simulink model "Closed_loop_Practical_BPS_LQR_Controller"  (R2023b)
settings: Solver=VariableStepAuto  StartTime=0.0  StopTime=10  RelTol=1e-3
undefined symbols (not defined in the file): A, B, C, Continuous, D, Discrete, Ke, Kr, Time
libraries: ctrlSharedLib x2, simulink_extras x1, simulink x1
settings Model: Creator=msdbg  LastModifiedBy=msdbg

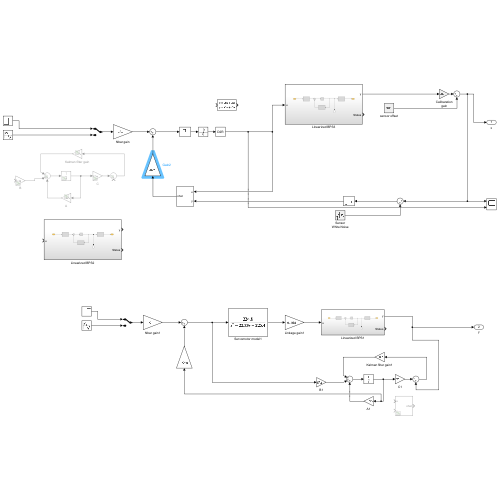
[thumbnail: Simulink's stored preview of the top-level diagram]
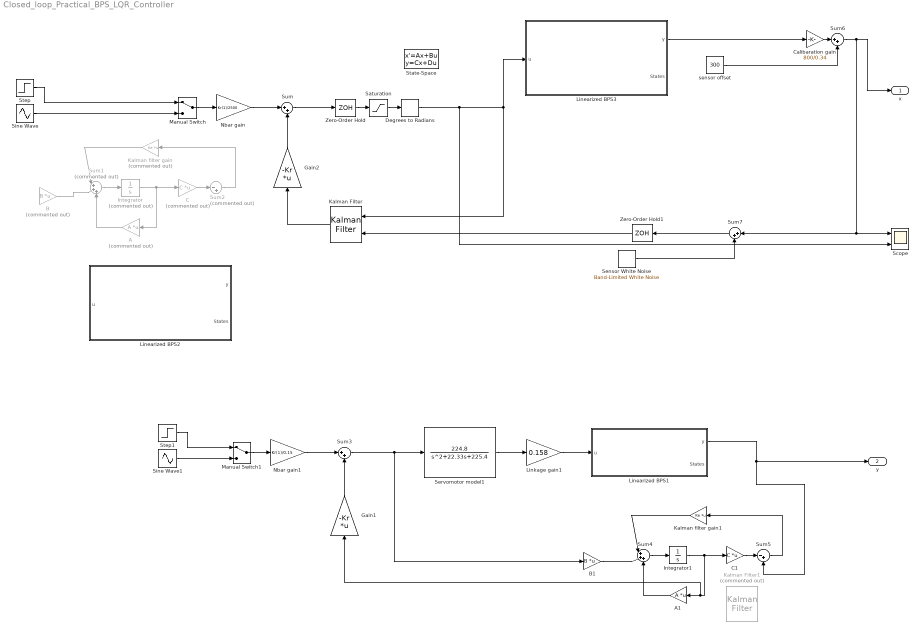
== system Closed_loop_Practical_BPS_LQR_Controller ==
  A : Gain  Commented=on  Gain=A  Multiplication=Matrix(K*u)
  A1 : Gain  Gain=A  Multiplication=Matrix(K*u)
  B : Gain  Commented=on  Gain=B  Multiplication=Matrix(K*u)
  B1 : Gain  Gain=B  Multiplication=Matrix(K*u)
  C : Gain  Commented=on  Gain=C  Multiplication=Matrix(K*u)
  C1 : Gain  Gain=C  Multiplication=Matrix(K*u)
  Calibaration gain : Gain  Gain=800/0.34
  Degrees to Radians : simulink_extras/Transformations/Degrees to Radians
  Gain1 : Gain  Gain=-Kr  Multiplication=Matrix(K*u)
  Gain2 : Gain  Gain=-Kr  Multiplication=Matrix(K*u)
  Integrator : Integrator  Commented=on
  Integrator1 : Integrator
  Kalman Filter : ctrlSharedLib/Kalman Filter  TimeDomain=Discrete-Time  UseCurrentEstimator=on  ModelSource=LTI State-Space Variable  ModelSourceVariable=DBPS  A=A  B=B  C=C  D=D  NumberOfStates=1  NumberOfInputs=1  NumberOfOutputs=1  InitialEstimateSource=Dialog  X0=0  P0=10  UseK=off  UseGH=off  NumberOfProcessNoiseInputs=1  G=1  TimeInvariantG=on  H=0  TimeInvariantH=on  Q=w  TimeInvariantQ=on  R=0.01  TimeInvariantR=on  N=0  TimeInvariantN=on  AddInputPort=on  AddEnablePort=off  OutputEstimatedY=off  OutputP=off  Ts=0.05
  Kalman Filter1 : ctrlSharedLib/Kalman Filter  Commented=on  TimeDomain=Continuous-Time  UseCurrentEstimator=on  ModelSource=LTI State-Space Variable  ModelSourceVariable=BPS  A=0.95  B=1  C=1  D=0  NumberOfStates=1  NumberOfInputs=1  NumberOfOutputs=1  InitialEstimateSource=Dialog  X0=0  P0=10  UseK=off  UseGH=off  NumberOfProcessNoiseInputs=1  G=1  TimeInvariantG=on  H=0  TimeInvariantH=on  Q=w  TimeInvariantQ=on  R=0.01  TimeInvariantR=on  N=0  TimeInvariantN=on  AddInputPort=on  AddEnablePort=off  OutputEstimatedY=off  OutputP=off  Ts=-1
  Kalman filter gain : Gain  Commented=on  Gain=Ke  Multiplication=Matrix(K*u)
  Kalman filter gain1 : Gain  Gain=Ke  Multiplication=Matrix(K*u)
  Linearized BPS1 : Subsystem
  Linearized BPS2 : Subsystem
  Linearized BPS3 : Subsystem
  Linkage gain1 : Gain  Gain=0.158
  Manual Switch : ManualSwitch
  Manual Switch1 : ManualSwitch
  Nbar gain : Gain  Gain=Kr(1)/2500
  Nbar gain1 : Gain  Gain=Kr(1)/0.15
  Saturation : Saturate  UpperLimit=90  LowerLimit=-90
  Scope : Scope  NumInputPorts=2
  Sensor White Noise : simulink/Sources/Band-Limited White Noise  Cov=[0.7]  Ts=0.1  seed=[23341]
  Servomotor model1 : TransferFcn  Numerator=[224.8]  Denominator=[1 22.33 225.4]
  Sine Wave : Sin  SampleTime=0
  Sine Wave1 : Sin  SampleTime=0
  State-Space : StateSpace  A=A  B=B  C=C  D=D  InitialCondition=0
  Step : Step  Time=0  After=550  SampleTime=0
  Step1 : Step  Time=0  SampleTime=0
  Sum{,3,6..7} (4 alike) : Sum  Inputs=|++
  Sum1 : Sum  Commented=on  Inputs=|+++
  Sum2 : Sum  Commented=on  Inputs=|-+
  Sum4 : Sum  Inputs=|+++
  Sum5 : Sum  Inputs=|-+
  Zero-Order Hold : ZeroOrderHold  SampleTime=0.05
  Zero-Order Hold1 : ZeroOrderHold  SampleTime=0.05
  sensor offset : Constant  Value=300
  x : Outport
  y : Outport  Port=2
  wires:
  Sum2/1 -> Kalman filter gain/1
  A/1 -> Sum1/3
  Integrator/1 -> A/1, C/1
  Gain2/1 -> Sum/2
  Sine Wave/1 -> Manual Switch/2
  Step/1 -> Manual Switch/1
  Kalman filter gain/1 -> Sum1/1
  Linkage gain1/1 -> Linearized BPS1/1(u)
  C/1 -> Sum2/1
  B/1 -> Sum1/2
  Sum1/1 -> Integrator/1
  Nbar gain1/1 -> Sum3/1
  Step1/1 -> Manual Switch1/1
  Kalman filter gain1/1 -> Sum4/1
  C1/1 -> Sum5/1
  Gain1/1 -> Sum3/2
  Integrator1/1 -> Gain1/1, A1/1, C1/1
  Linearized BPS1/1(y) -> Sum5/2, y/1
  Servomotor model1/1 -> Linkage gain1/1
  Sum3/1 -> B1/1, Servomotor model1/1
  Manual Switch1/1 -> Nbar gain1/1
  Sine Wave1/1 -> Manual Switch1/2
  Sum5/1 -> Kalman filter gain1/1
  B1/1 -> Sum4/2
  A1/1 -> Sum4/3
  Sum4/1 -> Integrator1/1
  Kalman Filter/1 -> Gain2/1
  Manual Switch/1 -> Nbar gain/1
  Calibaration gain/1 -> Sum6/1
  sensor offset/1 -> Sum6/2
  Sensor White Noise/1 -> Sum7/2
  Linearized BPS3/1(y) -> Calibaration gain/1
  Sum7/1 -> Zero-Order Hold1/1
  Nbar gain/1 -> Sum/1
  Sum6/1 -> Sum7/1, Scope/1, x/1
  Zero-Order Hold/1 -> Saturation/1
  Zero-Order Hold1/1 -> Kalman Filter/2
  Saturation/1 -> Degrees to Radians/1
  Degrees to Radians/1 -> Scope/2, Kalman Filter/1, Linearized BPS3/1(u)
  Sum/1 -> Zero-Order Hold/1

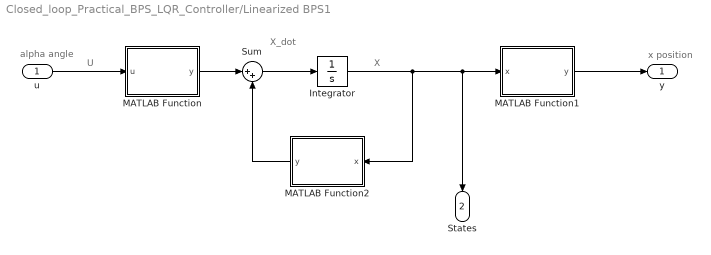
== system Closed_loop_Practical_BPS_LQR_Controller/Linearized BPS1 ==
  note: x position
  note: alpha angle
  note: X
  note: X_dot
  note: U
  u : Inport
  Integrator : Integrator
  MATLAB Function : MATLAB Function  TreatAsAtomicUnit=on
  MATLAB Function1 : MATLAB Function  TreatAsAtomicUnit=on
  MATLAB Function2 : MATLAB Function  TreatAsAtomicUnit=on
  Sum : Sum  Inputs=|++
  y : Outport
  States : Outport  Port=2
  wires:
  Sum/1 -> Integrator/1
  Integrator/1 -> MATLAB Function2/1(x), States/1, MATLAB Function1/1(x)
  MATLAB Function/1(y) -> Sum/1
  u/1 -> MATLAB Function/1(u)
  MATLAB Function2/1(y) -> Sum/2
  MATLAB Function1/1(y) -> y/1

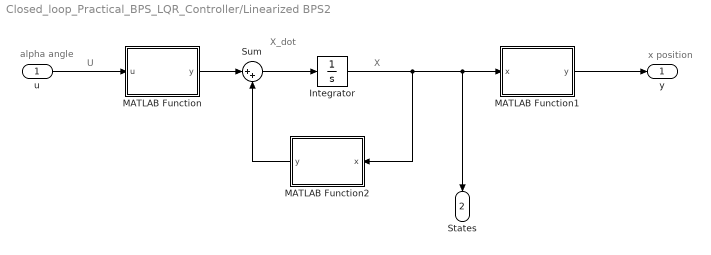
== system Closed_loop_Practical_BPS_LQR_Controller/Linearized BPS2 ==
  note: x position
  note: alpha angle
  note: X
  note: X_dot
  note: U
  u : Inport
  Integrator : Integrator
  MATLAB Function : MATLAB Function  TreatAsAtomicUnit=on
  MATLAB Function1 : MATLAB Function  TreatAsAtomicUnit=on
  MATLAB Function2 : MATLAB Function  TreatAsAtomicUnit=on
  Sum : Sum  Inputs=|++
  y : Outport
  States : Outport  Port=2
  wires:
  Sum/1 -> Integrator/1
  Integrator/1 -> MATLAB Function2/1(x), States/1, MATLAB Function1/1(x)
  MATLAB Function/1(y) -> Sum/1
  u/1 -> MATLAB Function/1(u)
  MATLAB Function2/1(y) -> Sum/2
  MATLAB Function1/1(y) -> y/1

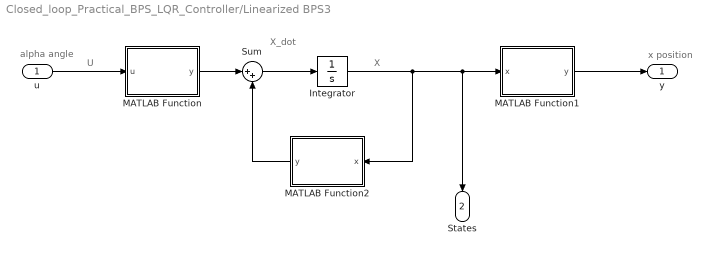
== system Closed_loop_Practical_BPS_LQR_Controller/Linearized BPS3 ==
  note: U
  note: X_dot
  note: X
  note: alpha angle
  note: x position
  u : Inport
  Integrator : Integrator
  MATLAB Function : MATLAB Function  TreatAsAtomicUnit=on
  MATLAB Function1 : MATLAB Function  TreatAsAtomicUnit=on
  MATLAB Function2 : MATLAB Function  TreatAsAtomicUnit=on
  Sum : Sum  Inputs=|++
  y : Outport
  States : Outport  Port=2
  wires:
  MATLAB Function1/1(y) -> y/1
  MATLAB Function2/1(y) -> Sum/2
  u/1 -> MATLAB Function/1(u)
  MATLAB Function/1(y) -> Sum/1
  Integrator/1 -> MATLAB Function1/1(x), States/1, MATLAB Function2/1(x)
  Sum/1 -> Integrator/1

== matlab function Closed_loop_Practical_BPS_LQR_Controller/Linearized BPS2/MATLAB Function1 ==
  data: x input size=[4 1]; y output
function y = C(x)

y = [1 0 0 0]*x;

== matlab function Closed_loop_Practical_BPS_LQR_Controller/Linearized BPS2/MATLAB Function2 ==
  data: x input size=[4 1]; y output size=[4 1]
function y = A(x)

y = [0 1 0 0; 0 0 -5/7*9.81 0; 0 0 0 1; 0 0 -225.4 -22.33]*x;

== matlab function Closed_loop_Practical_BPS_LQR_Controller/Linearized BPS1/MATLAB Function ==
  data: u input; y output
function y = B(u)

y = [0; 5/7*9.81].*u;

== matlab function Closed_loop_Practical_BPS_LQR_Controller/Linearized BPS1/MATLAB Function1 ==
  data: x input size=[2 1]; y output
function y = C(x)

y = [1 0]*x;

== matlab function Closed_loop_Practical_BPS_LQR_Controller/Linearized BPS1/MATLAB Function2 ==
  data: x input size=[2 1]; y output size=[2 1]
function y = A(x)

y = [0 1 ; 0 0]*x;

== matlab function Closed_loop_Practical_BPS_LQR_Controller/Linearized BPS3/MATLAB Function ==
  data: u input; y output
function y = B(u)

y = [0; 0; 0; 225.4].*u;

== matlab function Closed_loop_Practical_BPS_LQR_Controller/Linearized BPS3/MATLAB Function1 ==
  data: x input size=[4 1]; y output
function y = C(x)

y = [1 0 0 0]*x;

== matlab function Closed_loop_Practical_BPS_LQR_Controller/Linearized BPS3/MATLAB Function2 ==
  data: x input size=[4 1]; y output size=[4 1]
function y = A(x)

y = [0 1 0 0; 0 0 -5/7*9.81 0; 0 0 0 1; 0 0 -225.4 -22.33]*x;

== matlab function Closed_loop_Practical_BPS_LQR_Controller/Linearized BPS2/MATLAB Function ==
  data: u input; y output
function y = B(u)

y = [0; 0; 0; 225.4].*u;
